simulink model "TEST_LIDAR"  (R2022b)
settings: Solver=FixedStepAuto  StartTime=0.0  StopTime=inf  FixedStep=1e-3  RelTol=1e-3  EnableMultiTasking=on
model workspace (MAT data in the model file):
  SL_ROS_VariableLengthArrays_MaxSizes : object (value not decoded)
values from neighbouring files (symbols this model uses):
  data = theClient.GetLastFrameOfData()    [FuncMotive.m]
undefined symbols (not defined in the file or in its folder): angular, carstamp, CIRCUIT, CLTF_DAMP, CLTF_FREQ, CLTF_GAIN, CONTROL, CONTROL_INI, DiscIntNeverNeededParam, INPUT, linear, MCP3201, MD25, MODEL, MODEL_INI, mpcstate, MPU60X0, MPU9250, MSG, NAV_MPC_CONTROL, OUTPUT, RCRX, SAMPLING_TIME, SYSID_INPUT, VL6180X
libraries: raspberrypiCommlib x160, simulink x89, raspberrypiNetworklib x22, ros2lib x14, dspsigattribs x14, embedlinuxBasiclib x12, ctrlSharedLib x2, mpclib x1, vrlib x1, sldrtlib x1
(part 19 of 19)

== matlab function TEST_LIDAR/CONTROL/LOCAL TARGETS/WFL TARGETS/ PULSE GENERATION ==
  data: CONTROL input Bus: CONTROL_Bus; WALL_DIST_REF output
function WALL_DIST_REF = PULSE_GEN(CONTROL)
    
persistent TIMER initialize
if isempty(initialize)
    TIMER = 0;
    initialize = 1;
end

% SAMPLING TIME
SAMPLING_TIME = CONTROL.PARAM.SAMPLING_TIME; % s

%% OPERATION MODE
% / 0. BOOTING   / 1. SENSOR CALIBRATION / 2. READY
% / 3. OPEN LOOP / 4. ATTITUDE / 5. VELOCITY / 6. NAVIGATION / 
% / 7. WALL FOLLOWER / 8. WALL-FOLLOWER COMPETITION / 
% / 9. NAVIGATION COMPETITION / 10. STOP
CURRENT_STATUS = CONTROL.STATE.CURRENT_STATUS_SYS;
PREVIOUS_STATUS = CONTROL.STATE.PREVIOUS_STATUS;

if (CURRENT_STATUS == 7) && (PREVIOUS_STATUS == 7)   
    if TIMER > 15
        WALL_DIST_REF = 0.1;
    elseif TIMER < 5
        WALL_DIST_REF = 0.1;
        TIMER = TIMER + SAMPLING_TIME;
    else % 5 <= TIMER <= 15
        WALL_DIST_REF = 0.125;
        TIMER = TIMER + SAMPLING_TIME;
    end
else
    WALL_DIST_REF = 0.1;
    TIMER = 0;
end

== matlab function TEST_LIDAR/CONTROL/SYSTEM IDENTIFICATION/Second-order equation ==
  data: b input; r1 output; c input; r2 output
function [r1,r2] = sol_2ord_eq(b,c)
r1 = (-b+sqrt(abs(b^2-4*c)))/2;
r2 = (-b-sqrt(abs(b^2-4*c)))/2;
return

== matlab function TEST_LIDAR/SIMULATION/READ IMU/IMU CALIBRATION ==
  data: CONTROL_IN input; ACCEL input; ACCEL_FILT input; ACCEL_MEAN input; ACCEL_MEAN_FILT input; GYRO input; GYRO_FILT input; GYRO_MEAN input; GYRO_MEAN_FILT input; ACCEL_CALIB input; ALFA_CALIB input; ACCEL_OFFS_IN input; GYRO_OFFS_IN input; CONTROL output Bus: CONTROL_Bus; ACCEL_OFFS_OUT output; GYRO_OFFS_OUT output; GRAVITY_VECTOR input
function [CONTROL,ACCEL_OFFS_OUT,GYRO_OFFS_OUT] = IMU_CALIBRATION(CONTROL_IN,...
                       ACCEL,ACCEL_FILT,ACCEL_MEAN,ACCEL_MEAN_FILT,...
                       GYRO,GYRO_FILT,GYRO_MEAN,GYRO_MEAN_FILT,...
                       ACCEL_CALIB,ALFA_CALIB,ACCEL_OFFS_IN,GYRO_OFFS_IN,GRAVITY_VECTOR)
                        
%--------------------------------------------------------------
% COPY CONTROL BUS
%--------------------------------------------------------------
CONTROL = CONTROL_IN;

%--------------------------------------------------------------
% IMU ORIENTATION
%--------------------------------------------------------------
% ACCEL = [1 0 0 ; 0 1 0 ; 0 0 1]*ACCEL;
% GYRO = [1 0 0 ; 0 1 0 ; 0 0 1]*GYRO;
ACCEL_MEAN = [1 0 0 ; 0 1 0 ; 0 0 1]*ACCEL_MEAN;
GYRO_MEAN = [1 0 0 ; 0 1 0 ; 0 0 1]*GYRO_MEAN;
% ACCEL_FILT = [1 0 0 ; 0 1 0 ; 0 0 1]*ACCEL_FILT;
% GYRO_FILT = [1 0 0 ; 0 1 0 ; 0 0 1]*GYRO_FILT;
ACCEL_MEAN_FILT = [1 0 0 ; 0 1 0 ; 0 0 1]*ACCEL_MEAN_FILT;
GYRO_MEAN_FILT = [1 0 0 ; 0 1 0 ; 0 0 1]*GYRO_MEAN_FILT;

%--------------------------------------------------------------
% CALIBRATION 
%--------------------------------------------------------------
if CONTROL.STATE.CURRENT_STATUS_SYS == 1  % CALIBRATION ENABLED
    if ACCEL_CALIB % ACCELEROMETER CALIBRATION ENABLED
        ACCEL_OFFS_OUT = ALFA_CALIB*ACCEL_OFFS_IN + (1-ALFA_CALIB)*(ACCEL_MEAN_FILT-GRAVITY_VECTOR);
    else
        ACCEL_OFFS_OUT = ACCEL_OFFS_IN;
    end
    GYRO_OFFS_OUT  = ALFA_CALIB*GYRO_OFFS_IN  + (1-ALFA_CALIB)*GYRO_MEAN_FILT;
else % END OF CALIBRATION
    if CONTROL.STATE.VEHICLE_MODE == 1
        ACCEL_OFFS_OUT = zeros(3,1);
    else
        ACCEL_OFFS_OUT = ACCEL_OFFS_IN;
    end   
    GYRO_OFFS_OUT  = GYRO_OFFS_IN;
    % ACCEL = ACCEL - ACCEL_OFFS_OUT;
    % GYRO = GYRO - GYRO_OFFS_OUT;
    ACCEL_MEAN = ACCEL_MEAN - ACCEL_OFFS_OUT;
    GYRO_MEAN = GYRO_MEAN - GYRO_OFFS_OUT;
    % ACCEL_FILT = ACCEL_FILT - ACCEL_OFFS_OUT;
    % GYRO_FILT = GYRO_FILT - GYRO_OFFS_OUT;
    ACCEL_MEAN_FILT = ACCEL_MEAN_FILT - ACCEL_OFFS_OUT;
    GYRO_MEAN_FILT = GYRO_MEAN_FILT - GYRO_OFFS_OUT;
end

%--------------------------------------------------------------
% IMU BUS UPDATE
%--------------------------------------------------------------
CONTROL.INPUT.IMU_ACCEL_MEAN = ACCEL_MEAN;
CONTROL.INPUT.IMU_GYRO_MEAN = GYRO_MEAN;
CONTROL.INPUT.IMU_ACCEL_MEAN_FILT = ACCEL_MEAN_FILT;
CONTROL.INPUT.IMU_GYRO_MEAN_FILT = GYRO_MEAN_FILT;

return
